simulink model "EV_1spd_4AUB10"  (R2021a)
settings: Solver=VariableStepAuto  StartTime=0.0  StopTime=1800  RelTol=1e-3
values from neighbouring files (symbols this model uses):
  e_gb = 0.97    [run_EV_PT_1spd.m]
  g1 = x(2)    [run_EV_PT_1spd.m]
  J_em = 0.1    [run_EV_PT_1spd.m]
  lambda = 1.05    [run_EV_PT_1spd.m]
  Paux = 0    [run_EV_PT_1spd.m]
  Ploss = 100    [run_EV_PT_1spd.m]
  scale_EM = x(4)    [run_EV_PT_1spd.m]
  wem_min = 1    [run_EV_PT_1spd.m]
undefined symbols (not defined in the file or in its folder): eta_EM_map, T_EM_max, w_EM_row, w_EM_upper
libraries: qss_tb_library_4AUB10 x5
settings Model: Creator=dadikozyanaa  LastModifiedBy=20203160

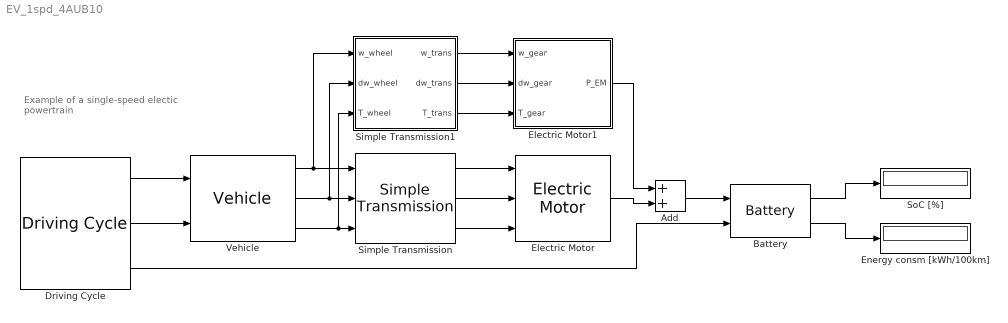
== system EV_1spd_4AUB10 ==
  note: Example of a single-speed electic powertrain
  Add : Sum
  Battery : qss_tb_library_4AUB10/Energy Buffer/Battery  init_SoC=init_SoC  bt_Np=10  bt_Ns=30
  Driving Cycle : qss_tb_library_4AUB10/Driving Cycle/Driving Cycle  Tag=cycle  cyclenr=Europe: WLTP Class 3  stepsize=1  autostop=on
  Electric Motor : qss_tb_library_4AUB10/Energy Converter/Electric Motor  scale_EM=scale_EM  theta_EM=J_em  P_aux=Paux
  Electric Motor1 : Subsystem  AncestorBlock=qss_tb_library_4AUB10/Energy Converter/Electric Motor  mask(Electric Motor){scale_EM=scale_EM, theta_EM=J_em, P_aux=Paux}
      mask prompts: scale_EM "Motor scaling factor [-]"; theta_EM "Motor inertia [kg*m2]"; P_aux "Power required by auxiliaries [W]"
      mask help:
      | This block simulates the behaviour of an electric motor. The block is based on an efficiency map.
      |
      | Input:
      | =====
      | 	w_gear		Speed of the fly wheel [rad/s]
      | 	dw_gear	Acceleration of the fly wheel [rad/s^2]
      | 	T_gear		Torque on the fly wheel [Nm]
      |
      | Output:
      | ======
      | 	P_EM		Power produced by the electric motor [W]
      mask init:
      | init_EM;
  Energy consm [kWh/100km] : Display
  Simple Transmission : qss_tb_library_4AUB10/Gear System/Simple Transmission  Tag=simple transmission  gear_ratio=g1  e_GT=e_gb  P_GT0=Ploss  w_wheel_min=wem_min
  Simple Transmission1 : Subsystem  Tag=simple transmission  AncestorBlock=qss_tb_library_4AUB10/Gear System/Simple Transmission  mask(Simple Transmission){gear_ratio=g1, e_GT=e_gb, P_GT0=Ploss, w_wheel_min=wem_min}
      mask prompts: gear_ratio "Gear ratio [-]"; e_GT "Efficiency [-]"; P_GT0 "Idling losses (friction) [W]"; w_wheel_min "Minimum wheel speed beyond which losses are generated [rad/s]"
      mask help:
      | This block simulates a transmission with a fixed gear ratio.
      |
      | Input:
      | =====
      | 	w_wheel	Speed of the wheel [rad/s]
      | 	dw_wheel	Acceleration of the wheel [rad/s^2]
      | 	T_wheel	Torque on the wheel [Nm]
      |
      | Output:
      | ======
      | 	w_trans		Speed of the fly wheel [rad/s]
      | 	dw_trans	Acceleration of the fly wheel [rad/s^2]
      | 	T_trans		Torque on the fly wheel [Nm]
      mask init:
      | init_transmission;
  SoC [%] : Display
  Vehicle : qss_tb_library_4AUB10/Vehicle/Vehicle  Tag=vehicle  m_f=mv  mt2m_f=lambda*100-100  A_f=Af  d_wheel=dw  cw=cd  mu=cr  f_r=f_r
  wires:
  Driving Cycle/1 -> Vehicle/1
  Driving Cycle/2 -> Vehicle/2
  Vehicle/1 -> Simple Transmission1/1(w_wheel), Simple Transmission/1
  Vehicle/2 -> Simple Transmission1/2(dw_wheel), Simple Transmission/2
  Vehicle/3 -> Simple Transmission1/3(T_wheel), Simple Transmission/3
  Simple Transmission/1 -> Electric Motor/1
  Simple Transmission/2 -> Electric Motor/2
  Simple Transmission/3 -> Electric Motor/3
  Electric Motor/1 -> Add/2
  Driving Cycle/3 -> Battery/2
  Battery/1 -> SoC [%]/1
  Battery/2 -> Energy consm [kWh/100km]/1
  Simple Transmission1/3(T_trans) -> Electric Motor1/3(T_gear)
  Simple Transmission1/2(dw_trans) -> Electric Motor1/2(dw_gear)
  Simple Transmission1/1(w_trans) -> Electric Motor1/1(w_gear)
  Electric Motor1/1(P_EM) -> Add/1
  Add/1 -> Battery/1

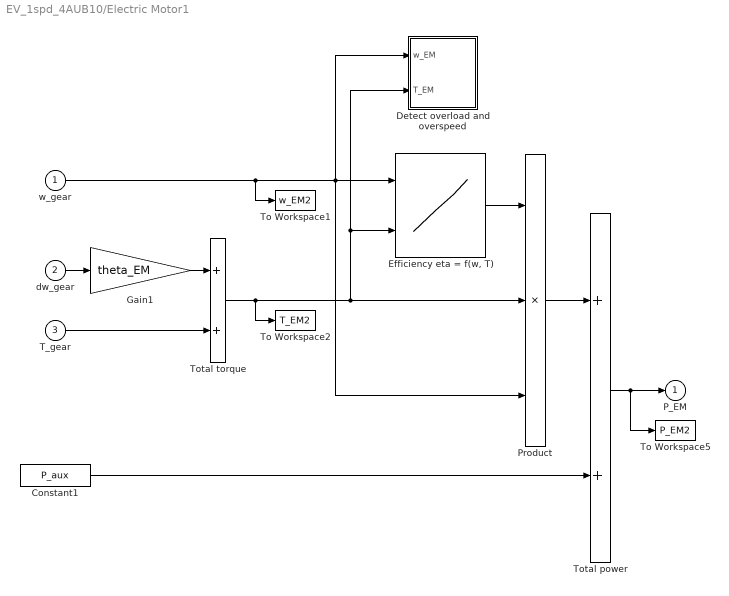
== system EV_1spd_4AUB10/Electric Motor1 ==
  w_gear : Inport
  dw_gear : Inport  Port=2
  T_gear : Inport  Port=3
  Constant1 : Constant  Value=P_aux
  Detect overload and overspeed : Subsystem
  "Efficiency eta = f(w, T)" : Lookup2D  RowIndex=w_EM_row  ColumnIndex=T_EM_col  Table=eta_EM_map
  Gain1 : Gain  Gain=theta_EM  SaturateOnIntegerOverflow=on  OutDataTypeStr=Inherit: Same as input  ParamDataTypeStr=Inherit: Same as input
  Product : Product  Inputs=3  InputSameDT=on  RndMeth=Zero  SaturateOnIntegerOverflow=on  OutDataTypeStr=Inherit: Same as first input
  To Workspace1 : ToWorkspace  VariableName=w_EM2  SampleTime=-1
  To Workspace2 : ToWorkspace  VariableName=T_EM2  SampleTime=-1
  To Workspace5 : ToWorkspace  VariableName=P_EM2  SampleTime=-1
  Total power : Sum  InputSameDT=on  SaturateOnIntegerOverflow=on  OutDataTypeStr=Inherit: Same as first input
  Total torque : Sum  InputSameDT=on  SaturateOnIntegerOverflow=on  OutDataTypeStr=Inherit: Same as first input
  P_EM : Outport  InitialOutput=0
  wires:
  Total power/1 -> To Workspace5/1, P_EM/1
  Product/1 -> Total power/1
  Constant1/1 -> Total power/2
  Total torque/1 -> To Workspace2/1, Product/2, "Efficiency eta = f(w, T)"/2, Detect overload and overspeed/2(T_EM)
  Gain1/1 -> Total torque/1
  T_gear/1 -> Total torque/2
  dw_gear/1 -> Gain1/1
  "Efficiency eta = f(w, T)"/1 -> Product/1
  w_gear/1 -> To Workspace1/1, Product/3, "Efficiency eta = f(w, T)"/1, Detect overload and overspeed/1(w_EM)

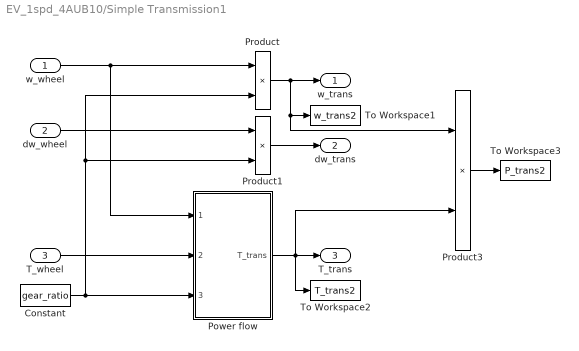
== system EV_1spd_4AUB10/Simple Transmission1 ==
  w_wheel : Inport
  dw_wheel : Inport  Port=2
  T_wheel : Inport  Port=3
  Constant : Constant  Value=gear_ratio
  Power flow : Subsystem
  Product : Product  InputSameDT=on  RndMeth=Zero  SaturateOnIntegerOverflow=on  OutDataTypeStr=Inherit: Same as first input
  Product1 : Product  InputSameDT=on  RndMeth=Zero  SaturateOnIntegerOverflow=on  OutDataTypeStr=Inherit: Same as first input
  Product3 : Product  InputSameDT=on  RndMeth=Zero  SaturateOnIntegerOverflow=on  OutDataTypeStr=Inherit: Same as first input
  To Workspace1 : ToWorkspace  VariableName=w_trans2  SampleTime=-1
  To Workspace2 : ToWorkspace  VariableName=T_trans2  SampleTime=-1
  To Workspace3 : ToWorkspace  VariableName=P_trans2  SampleTime=-1
  w_trans : Outport  InitialOutput=0
  dw_trans : Outport  Port=2  InitialOutput=0
  T_trans : Outport  Port=3  InitialOutput=0
  wires:
  Product3/1 -> To Workspace3/1
  w_wheel/1 -> Power flow/1(w_wheel), Product/1
  Constant/1 -> Product/2, Product1/2, Power flow/3(gear_ratio)
  T_wheel/1 -> Power flow/2(T_wheel)
  dw_wheel/1 -> Product1/1
  Product/1 -> Product3/1, To Workspace1/1, w_trans/1
  Product1/1 -> dw_trans/1
  Power flow/1(T_trans) -> Product3/2, To Workspace2/1, T_trans/1

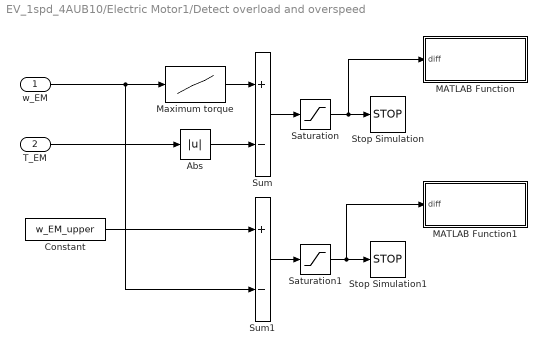
== system EV_1spd_4AUB10/Electric Motor1/Detect overload and overspeed ==
  w_EM : Inport
  T_EM : Inport  Port=2
  Abs : Abs  SaturateOnIntegerOverflow=on
  Constant : Constant  Value=w_EM_upper
  MATLAB Function : MATLAB Function  TreatAsAtomicUnit=on
  MATLAB Function1 : MATLAB Function  TreatAsAtomicUnit=on
  Maximum torque : Lookup  InputValues=w_EM_row  Table=T_EM_max  SaturateOnIntegerOverflow=on
  Saturation : Saturate  UpperLimit=0  LowerLimit=-inf
  Saturation1 : Saturate  UpperLimit=0  LowerLimit=-inf
  Stop Simulation : Stop
  Stop Simulation1 : Stop
  Sum : Sum  Inputs=+-  InputSameDT=on  SaturateOnIntegerOverflow=on  OutDataTypeStr=Inherit: Same as first input
  Sum1 : Sum  Inputs=+-  InputSameDT=on  SaturateOnIntegerOverflow=on  OutDataTypeStr=Inherit: Same as first input
  wires:
  Sum/1 -> Saturation/1
  w_EM/1 -> Maximum torque/1, Sum1/2
  T_EM/1 -> Abs/1
  Maximum torque/1 -> Sum/1
  Abs/1 -> Sum/2
  Saturation/1 -> Stop Simulation/1, MATLAB Function/1(diff)
  Constant/1 -> Sum1/1
  Sum1/1 -> Saturation1/1
  Saturation1/1 -> Stop Simulation1/1, MATLAB Function1/1(diff)

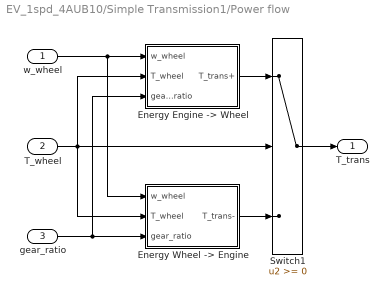
== system EV_1spd_4AUB10/Simple Transmission1/Power flow ==
  w_wheel : Inport
  T_wheel : Inport  Port=2
  gear_ratio : Inport  Port=3
  "Energy Engine -> Wheel" : Subsystem
  "Energy Wheel -> Engine" : Subsystem
  Switch1 : Switch  SaturateOnIntegerOverflow=on  InputSameDT=on
  T_trans : Outport  InitialOutput=0
  wires:
  Switch1/1 -> T_trans/1
  "Energy Engine -> Wheel"/1(T_trans+) -> Switch1/1
  T_wheel/1 -> Switch1/2, "Energy Engine -> Wheel"/2(T_wheel), "Energy Wheel -> Engine"/2(T_wheel)
  "Energy Wheel -> Engine"/1(T_trans-) -> Switch1/3
  gear_ratio/1 -> "Energy Engine -> Wheel"/3(gear_ratio), "Energy Wheel -> Engine"/3(gear_ratio)
  w_wheel/1 -> "Energy Engine -> Wheel"/1(w_wheel), "Energy Wheel -> Engine"/1(w_wheel)

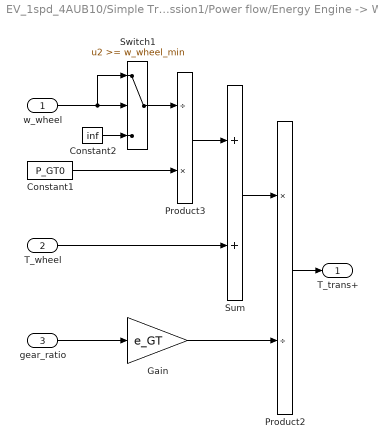
== system EV_1spd_4AUB10/Simple Transmission1/Power flow/Energy Engine -> Wheel ==
  w_wheel : Inport
  T_wheel : Inport  Port=2
  gear_ratio : Inport  Port=3
  Constant1 : Constant  Value=P_GT0
  Constant2 : Constant  Value=inf
  Gain : Gain  Gain=e_GT  SaturateOnIntegerOverflow=on  OutDataTypeStr=Inherit: Same as input  ParamDataTypeStr=Inherit: Same as input
  Product2 : Product  Inputs=*/  InputSameDT=on  RndMeth=Zero  SaturateOnIntegerOverflow=on  OutDataTypeStr=Inherit: Same as first input
  Product3 : Product  Inputs=/*  InputSameDT=on  RndMeth=Zero  SaturateOnIntegerOverflow=on  OutDataTypeStr=Inherit: Same as first input
  Sum : Sum  InputSameDT=on  SaturateOnIntegerOverflow=on  OutDataTypeStr=Inherit: Same as first input
  Switch1 : Switch  Threshold=w_wheel_min  SaturateOnIntegerOverflow=on  InputSameDT=on
  T_trans+ : Outport  InitialOutput=0
  wires:
  gear_ratio/1 -> Gain/1
  Constant1/1 -> Product3/2
  Switch1/1 -> Product3/1
  Constant2/1 -> Switch1/3
  w_wheel/1 -> Switch1/1, Switch1/2
  Sum/1 -> Product2/1
  Product2/1 -> T_trans+/1
  Gain/1 -> Product2/2
  Product3/1 -> Sum/1
  T_wheel/1 -> Sum/2

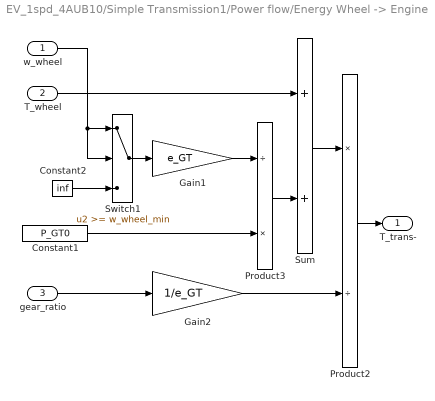
== system EV_1spd_4AUB10/Simple Transmission1/Power flow/Energy Wheel -> Engine ==
  w_wheel : Inport
  T_wheel : Inport  Port=2
  gear_ratio : Inport  Port=3
  Constant1 : Constant  Value=P_GT0
  Constant2 : Constant  Value=inf
  Gain1 : Gain  Gain=e_GT  SaturateOnIntegerOverflow=on  OutDataTypeStr=Inherit: Same as input  ParamDataTypeStr=Inherit: Same as input
  Gain2 : Gain  Gain=1/e_GT  SaturateOnIntegerOverflow=on  OutDataTypeStr=Inherit: Same as input  ParamDataTypeStr=Inherit: Same as input
  Product2 : Product  Inputs=*/  InputSameDT=on  RndMeth=Zero  SaturateOnIntegerOverflow=on  OutDataTypeStr=Inherit: Same as first input
  Product3 : Product  Inputs=/*  InputSameDT=on  RndMeth=Zero  SaturateOnIntegerOverflow=on  OutDataTypeStr=Inherit: Same as first input
  Sum : Sum  InputSameDT=on  SaturateOnIntegerOverflow=on  OutDataTypeStr=Inherit: Same as first input
  Switch1 : Switch  Threshold=w_wheel_min  SaturateOnIntegerOverflow=on  InputSameDT=on
  T_trans- : Outport  InitialOutput=0
  wires:
  Gain1/1 -> Product3/1
  Sum/1 -> Product2/1
  Product3/1 -> Sum/2
  Product2/1 -> T_trans-/1
  Gain2/1 -> Product2/2
  T_wheel/1 -> Sum/1
  Constant1/1 -> Product3/2
  Switch1/1 -> Gain1/1
  Constant2/1 -> Switch1/3
  gear_ratio/1 -> Gain2/1
  w_wheel/1 -> Switch1/2, Switch1/1

== matlab function EV_1spd_4AUB10/Electric Motor1/Detect overload and overspeed/MATLAB Function1 ==
  data: diff input
function error_EM_overspeed(diff)
if diff ~= 0
    disp("The EM is overspeeded!");
end
end

== matlab function EV_1spd_4AUB10/Electric Motor1/Detect overload and overspeed/MATLAB Function ==
  data: diff input
function error_EM_overload(diff)
if diff ~= 0
    disp("The EM is overloaded!");
end
end
